simulink model "CP_SFC_Lin_b_n9945008"  (R2018b)
settings: Solver=VariableStepAuto  StartTime=0.0  StopTime=5  FixedStep=0.02  RelTol=1e-3
values from neighbouring files (symbols this model uses):
  Ab = [ 0 ,        0           , 1 , 0 ... (first row only)    [CP_SFC_Lin_b_MainFile_n9945008.m]
  Bb = [0;0;1/Mc;1/(l*Mc)]    [CP_SFC_Lin_b_MainFile_n9945008.m]
  Cb = eye(4)    [CP_SFC_Lin_b_MainFile_n9945008.m]
  Db = zeros(4,1)    [CP_SFC_Lin_b_MainFile_n9945008.m]
  Kb = place(Ab,Bb, [-3,-4,-5,-6])    [CP_SFC_Lin_b_MainFile_n9945008.m]
  x0 = [0.2 20*pi/180 0 0]'    [CP_SFC_Lin_a_MainFile_n9945008.m]    (also in CP_SFC_Lin_b_MainFile_n9945008.m = [0.4 200*pi/180 0 0]')
settings Model: Creator=Cody  LastModifiedBy=Cody

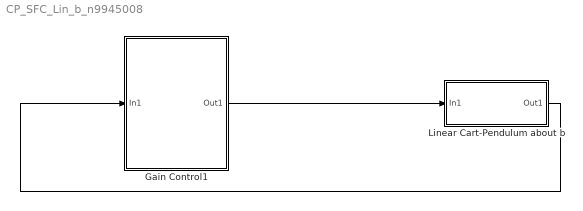
== system CP_SFC_Lin_b_n9945008 ==
  Gain Control1 : Subsystem
  "Linear Cart-Pendulum about b " : Subsystem
  wires:
  Gain Control1/1(Out1) -> "Linear Cart-Pendulum about b "/1(In1)
  "Linear Cart-Pendulum about b "/1(Out1) -> Gain Control1/1(In1)

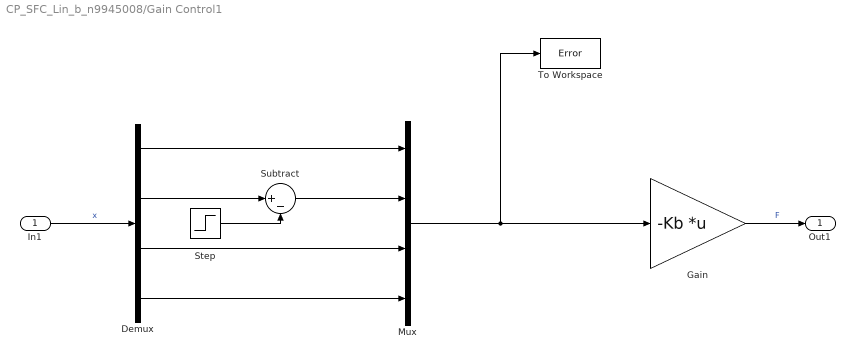
== system CP_SFC_Lin_b_n9945008/Gain Control1 ==
  In1 : Inport
  Demux : Demux
  Gain : Gain  Gain=-Kb  Multiplication=Matrix(K*u)
  Mux : Mux
  Step : Step  Time=0  After=pi  SampleTime=0
  Subtract : Sum  Inputs=|+-
  To Workspace : ToWorkspace  VariableName=Error  SampleTime=-1
      settings: Save2DSignal=2-D array (concatenate along first dimension)
  Out1 : Outport
  wires:
  Gain/1 -> Out1/1  "F"
  In1/1 -> Demux/1  "x"
  Mux/1 -> To Workspace/1, Gain/1
  Demux/1 -> Mux/1
  Demux/3 -> Mux/3
  Demux/4 -> Mux/4
  Subtract/1 -> Mux/2
  Demux/2 -> Subtract/1
  Step/1 -> Subtract/2

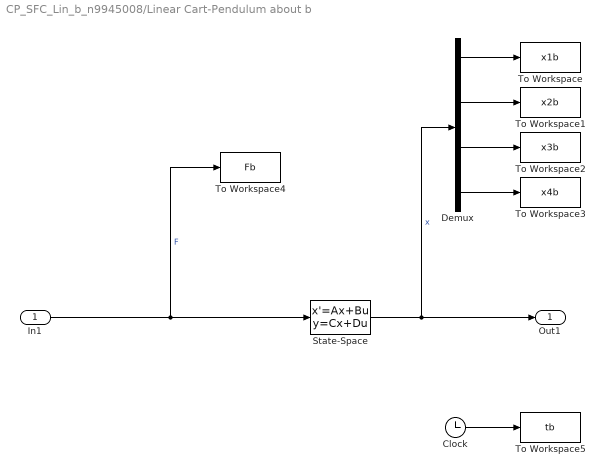
== system CP_SFC_Lin_b_n9945008/Linear Cart-Pendulum about b  ==
  In1 : Inport
  Clock : Clock
  Demux : Demux
  State-Space : StateSpace  A=Ab  B=Bb  C=Cb  D=Db  InitialCondition=x0
  To Workspace : ToWorkspace  VariableName=x1b  SampleTime=-1
      settings: Save2DSignal=2-D array (concatenate along first dimension)
  To Workspace1 : ToWorkspace  VariableName=x2b  SampleTime=-1
      settings: Save2DSignal=2-D array (concatenate along first dimension)
  To Workspace2 : ToWorkspace  VariableName=x3b  SampleTime=-1
      settings: Save2DSignal=2-D array (concatenate along first dimension)
  To Workspace3 : ToWorkspace  VariableName=x4b  SampleTime=-1
      settings: Save2DSignal=2-D array (concatenate along first dimension)
  To Workspace4 : ToWorkspace  VariableName=Fb  SampleTime=-1
      settings: Save2DSignal=2-D array (concatenate along first dimension)
  To Workspace5 : ToWorkspace  VariableName=tb  SampleTime=-1
      settings: Save2DSignal=2-D array (concatenate along first dimension)
  Out1 : Outport
  wires:
  In1/1 -> To Workspace4/1, State-Space/1  "F"
  State-Space/1 -> Demux/1, Out1/1  "x"
  Demux/1 -> To Workspace/1
  Demux/2 -> To Workspace1/1
  Demux/3 -> To Workspace2/1
  Demux/4 -> To Workspace3/1
  Clock/1 -> To Workspace5/1
